simulink model "AE_BoltEV_LMDI"  (R2026a)
settings: Solver=ode23t  StartTime=0  StopTime=1800  FixedStep=Ts  MaxStep=0.01  EnableMultiTasking=on
InitFcn:
  | AE_BoltEV_LMDI_Params;
undefined symbols (not defined in the file): id_map, iq_map, Is_map, n_loss_bp, P, P_cu_map, P_iron_map, T_loss_bp, Tmax, V_oc
libraries: nesl_utility x14, fl_lib x12, autolibshared x2, sdl_lib x2, autolibmappedmotor x1, sl_discontinuities x1
(part 3 of 3)

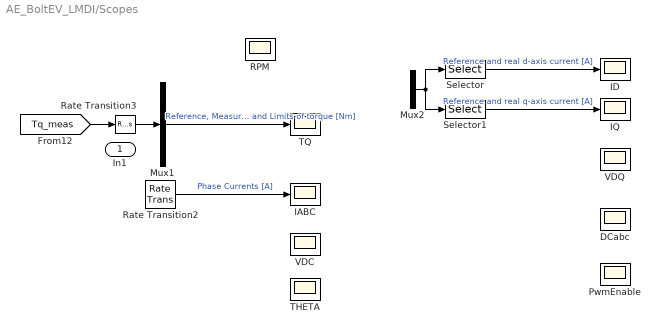
== system AE_BoltEV_LMDI/Scopes ==
  In1 : Inport
  DCabc : Scope
      settings: ActiveDisplayYMinimum=-1.2499998168622757  ActiveDisplayYMaximum=1.2499998168622755
  IABC : Scope
      settings: ActiveDisplayYMinimum=-1043.3720636046316  ActiveDisplayYMaximum=1044.7685894372053  DataLoggingVariableName=ScopeData5
  ID : Scope
      settings: ActiveDisplayYMinimum=-578.40556023238867  ActiveDisplayYMaximum=91.835041505026354  DataLoggingSaveFormat=Array
  IQ : Scope
      settings: ActiveDisplayYMinimum=-1  ActiveDisplayYMaximum=1  DataLoggingVariableName=ScopeData2  DataLoggingSaveFormat=Array
  Mux1 : Mux  Inputs=3
  Mux2 : Mux  Inputs=2
  PwmEnable : Scope
      settings: ActiveDisplayYMinimum=-0.12499999999999997  ActiveDisplayYMaximum=1.125  DataLoggingSaveFormat=Array
  RPM : Scope
      settings: ActiveDisplayYMinimum=-1  ActiveDisplayYMaximum=1
  Rate Transition2 : RateTransition  OutPortSampleTime=1e-4
  Rate Transition3 : RateTransition
  Selector : Selector  InputPortWidth=4  IndexOptions=Index vector (dialog)  Indices=[1 3]  OutputSizes=1
  Selector1 : Selector  InputPortWidth=4  IndexOptions=Index vector (dialog)  Indices=[2 4]  OutputSizes=1
  THETA : Scope
      settings: ActiveDisplayYMinimum=-0.78539816324069045  ActiveDisplayYMaximum=7.0685834691662164  DataLoggingVariableName=ScopeData7
  TQ : Scope
      settings: ActiveDisplayYMinimum=-34.876030026674364  ActiveDisplayYMaximum=3.8751144474082619  DataLoggingVariableName=ScopeData2
  VDC : Scope
      settings: ActiveDisplayYMinimum=-42.2212392731809  ActiveDisplayYMaximum=416.66871284749823  DataLoggingVariableName=ScopeData6
  VDQ : Scope
      settings: ActiveDisplayYMinimum=-252.94313596426539  ActiveDisplayYMaximum=264.44118716095903  DataLoggingVariableName=ScopeData8
  wires:
  Mux1/1 -> TQ/1  "Reference, Measured, Estim and Limits of torque [Nm]"
  Rate Transition2/1 -> IABC/1  "Phase Currents [A]"
  Selector1/1 -> IQ/1  "Reference and real q-axis current [A]"
  Selector/1 -> ID/1  "Reference and real d-axis current [A]"
  Mux2/1 -> Selector1/1, Selector/1
  [Tq_meas] -> Rate Transition3/1
  Rate Transition3/1 -> Mux1/2

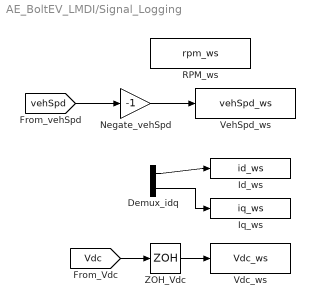
== system AE_BoltEV_LMDI/Signal_Logging ==
  Demux_idq : Demux  Outputs=2
  Id_ws : ToWorkspace  VariableName=id_ws  SampleTime=0.1
      settings: Decimation=100
  Iq_ws : ToWorkspace  VariableName=iq_ws  SampleTime=0.1
      settings: Decimation=100
  Negate_vehSpd : Gain  Gain=-1
  RPM_ws : ToWorkspace  VariableName=rpm_ws  SampleTime=0.1
      settings: Decimation=100
  Vdc_ws : ToWorkspace  VariableName=Vdc_ws  SampleTime=0.1
  VehSpd_ws : ToWorkspace  VariableName=vehSpd_ws  SampleTime=0.1
      settings: Decimation=2000
  ZOH_Vdc : ZeroOrderHold  SampleTime=0.01
  wires:
  Demux_idq/1 -> Id_ws/1
  [vehSpd] -> Negate_vehSpd/1
  ZOH_Vdc/1 -> Vdc_ws/1
  Demux_idq/2 -> Iq_ws/1
  [Vdc] -> ZOH_Vdc/1
  Negate_vehSpd/1 -> VehSpd_ws/1

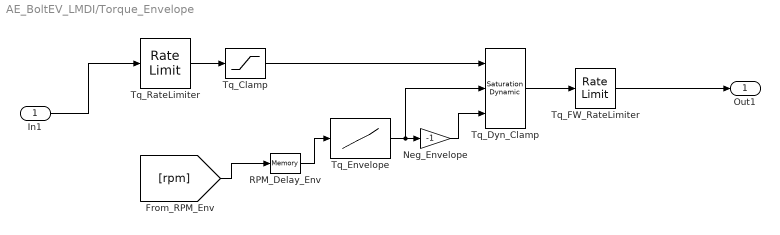
== system AE_BoltEV_LMDI/Torque_Envelope ==
  In1 : Inport
  Neg_Envelope : Gain  Gain=-1
  RPM_Delay_Env : Memory
  Tq_Clamp : Saturate  UpperLimit=Tmax  LowerLimit=-Tmax
  Tq_Dyn_Clamp : sl_discontinuities/Saturation Dynamic  OutMin=[]  OutMax=[]  OutDataTypeStr=Inherit: Same as second input  OutDataType=fixdt(1, 16)  OutScaling=2^-10  DoSatur=off
      settings: LibrarySourceBlock=|
      | simulink/Discontinuities/Saturation
      | Dynamic
  Tq_Envelope : Lookup_n-D  NumberOfTableDimensions=1  BreakpointsForDimension1=[0 1 3500 4400 5000 5500 6000 6500 7000 7500 8000 8800]  Table=[360 360 360 325 286 260 238 220 204 191 179 162]  ExtrapMethod=Clip  InternalRulePriority=Speed  RndMeth=Simplest
  Tq_FW_RateLimiter : RateLimiter  RisingSlewLimit=2000  FallingSlewLimit=-2000  SampleTimeMode=inherited
  Tq_RateLimiter : RateLimiter  RisingSlewLimit=1000  FallingSlewLimit=-1000  SampleTimeMode=inherited
  Out1 : Outport
  wires:
  In1/1 -> Tq_RateLimiter/1
  [rpm] -> RPM_Delay_Env/1
  RPM_Delay_Env/1 -> Tq_Envelope/1
  Tq_RateLimiter/1 -> Tq_Clamp/1
  Neg_Envelope/1 -> Tq_Dyn_Clamp/3
  Tq_Dyn_Clamp/1 -> Tq_FW_RateLimiter/1
  Tq_FW_RateLimiter/1 -> Out1/1
  Tq_Clamp/1 -> Tq_Dyn_Clamp/1
  Tq_Envelope/1 -> Tq_Dyn_Clamp/2, Neg_Envelope/1

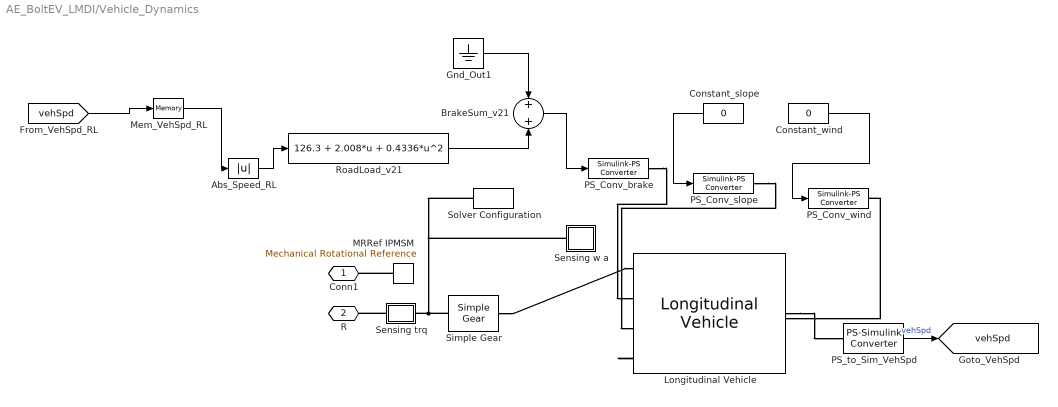
== system AE_BoltEV_LMDI/Vehicle_Dynamics ==
  Abs_Speed_RL : Abs  SaturateOnIntegerOverflow=off
  BrakeSum_v21 : Sum
  Constant_slope : Constant  Value=0
  Constant_wind : Constant  Value=0
  Gnd_Out1 : Ground
  Longitudinal Vehicle : sdl_lib/Tires & Vehicles/Longitudinal Vehicle  vehParamType=sdl.enum.VehicleParameterizationType.Regular  M_vehicle=1705 kg  R_tireroll=0.317 m  C_tireroll=1e-6  C_airdrag=1e-6  A_front=2.37 m^2  A_rl=178 N  B_rl=3.024 N*s/m  C_rl=0.36988 N*s^2/m^2  g=9.81 m/s^2  V_1=0.3 m/s  w_1=0.01 rad/s  ShowBrakeIn=true  ShowSlopeIn=true  SlopeInputType=sdl.enum.VehicleLongitudinalRoadSlopeInputType.GradePercent  ShowWindIn=true  ShowGOut=false  air_density=1.225 kg/m^3  V_x_specify=off  V_x_priority=High  V_x=0 m/s  V_x_nominal_specify=off  V_x_nominal_value=1  V_x_nominal_unit=m/s  trq_specify=off  trq_priority=None  trq=0 N*m  trq_nominal_specify=off  trq_nominal_value=1  trq_nominal_unit=N*m  w_specify=off  w_priority=None  w=0 rad/s  w_nominal_specify=off  w_nominal_value=1  w_nominal_unit=rad/s
  MRRef IPMSM : fl_lib/Mechanical/Rotational Elements/Mechanical Rotational Reference
  Mem_VehSpd_RL : Memory
  PS_Conv_brake : nesl_utility/Simulink-PS Converter  PhysicalDomain=network_engine_domain  SubClassName=ps_input  LeftPortType=input  RightPortType=output  PseudoPeriodic=off  Frequencies=[]  NoiseDistribution=none  NoiseParameters=[]  Unit=N  AffineConversion=off  FilteringAndDerivatives=provide  SimscapeFilterOrder=1  InputFilterTimeConstant=0.001  UdotUserProvided=0
  PS_Conv_slope : nesl_utility/Simulink-PS Converter  PhysicalDomain=network_engine_domain  SubClassName=ps_input  LeftPortType=input  RightPortType=output  PseudoPeriodic=off  Frequencies=[]  NoiseDistribution=none  NoiseParameters=[]  Unit=rad  AffineConversion=off  FilteringAndDerivatives=provide  SimscapeFilterOrder=1  InputFilterTimeConstant=0.001  UdotUserProvided=0
  PS_Conv_wind : nesl_utility/Simulink-PS Converter  PhysicalDomain=network_engine_domain  SubClassName=ps_input  LeftPortType=input  RightPortType=output  PseudoPeriodic=off  Frequencies=[]  NoiseDistribution=none  NoiseParameters=[]  Unit=m/s  AffineConversion=off  FilteringAndDerivatives=provide  SimscapeFilterOrder=1  InputFilterTimeConstant=0.001  UdotUserProvided=0
  PS_to_Sim_VehSpd : nesl_utility/PS-Simulink Converter  PhysicalDomain=network_engine_domain  SubClassName=ps_output  LeftPortType=input  RightPortType=output  PseudoPeriodic=off  Frequencies=[]  VectorFormat=inherit  Unit=m/s  AffineConversion=off
  RoadLoad_v21 : Fcn  Expr=126.3 + 2.008*u + 0.4336*u^2
  Sensing trq : Subsystem
      mask Display: disp('trq')
  Sensing w a : Subsystem
      mask Display: disp('w,a')
  Simple Gear : sdl_lib/Gears/Simple Gear  ratio=7.05  rotation_direction=sdl.enum.shaftOutputDirection.opposite  friction_model=sdl.enum.gear_efficiencies_load.constant  T_noload=0 N*m  T_nom=5 N*m  efficiency_nom=0.97  efficiency=gear_eff  temperature_TLU=[280, 300, 320] K  load_TLU=[1, 5, 10] N*m  efficiency_TLU=[.95, .9, .85]  efficiency_TLU2=[.85, .8, .75; .95, .9, .85; .85, .8, .7]  w_thr=0.01 rad/s  pwr_thr=0.001 W  enable_backlash=false  hardstop_model=simscape.enum.hardstop.smooth  backlash_distance=1e-3 mm  r_base=0.1 m  transition=1e-4 mm  backlash_stiffness=1e6 N/m  backlash_damping=1e3 N*s/m  coeff_rest=0.7  v_tol=0.001 m/s  f_tol=0.001 N  tau=0.1 s  mu_visc=[0 0] N*m*s/rad  thermal_mass=50 J/K  temperature_specify=off  temperature_priority=High  temperature=300 K  temperature_nominal_specify=off  temperature_nominal_value=1  temperature_nominal_unit=K  x_backlash_specify=off  x_backlash_priority=None  x_backlash=0 mm  x_backlash_nominal_specify=off  x_backlash_nominal_value=1  x_backlash_nominal_unit=mm  f_hardstop_specify=off  f_hardstop_priority=None  f_hardstop=0 N  f_hardstop_nominal_specify=off  f_hardstop_nominal_value=1  f_hardstop_nominal_unit=N  v_backlash_specify=off  v_backlash_priority=None  v_backlash=0 m/s  v_backlash_nominal_specify=off  v_backlash_nominal_value=1  v_backlash_nominal_unit=m/s
  Solver Configuration : nesl_utility/Solver Configuration  PhysicalDomain=network_engine_domain  SubClassName=solver  LeftPortType=input  RightPortType=generic  Tones=[]  Harmonics=[]  SimulateNoise=off  Profile=off  UseLocalSampling=off  EnableSwitchedLinearOptims=on  FrequencyDomain=off  UseCCode=off  RelTol=0.001  AbsTol=1e-06  MinStep=1e-09  ToWorkspace=off  RevertToSquareIcSolve=off  NumHomotopyIterations=100  PhasorMode=off  PhasorModeNumHarmonics=1  ConsistencySolver=NEWTON_FTOL  CanonicalOrdering=UNORDERED  OptimizeIntermediates=UNOPTIMIZED  IndexReductionMethod=DerivativeReplacement  DoDC=off  ResidualTolerance=1e-9  ConsistencyTolSource=GLOBAL  ConsistencyAbsTol=0.001  ConsistencyRelTol=0.001  ConsistencyTolFactor=0.001  UseLocalSolver=on  LocalSolverChoice=NE_BACKWARD_EULER_ADVANCER  ResolveIndetEquations=on  FunctionEvalNumThread=1  LocalSolverSampleTime=Ts  DoFixedCost=on  MaxNonlinIter=5  MaxModeIter=2  ComputeImpulses=off  ImpulseIterations=1  LinearAlgebra=auto  LinearAlgebraNumThread=0  EquationFormulation=NE_TIME_EF  DelaysMemoryBudget=1024  AutomaticFiltering=on  FilteringTimeConstant=0.001  PartitionStorageMethod=AS_NEEDED  PartitionMemoryBudget=1024  PartitionMethod=FAST  MultibodyUseLocalSolver=off  MultibodyLocalSolverChoice=ODE1  MultibodyLocalSolverSampleTime=0.001
  Conn1 : PMIOPort  Side=Left
  R : PMIOPort  Port=2  Side=Left
  tag scope: vehSpd=global
  wires:
  PS_to_Sim_VehSpd/1 -> [vehSpd]  "vehSpd"
  Constant_slope/1 -> PS_Conv_slope/1
  Constant_wind/1 -> PS_Conv_wind/1
  Abs_Speed_RL/1 -> RoadLoad_v21/1
  RoadLoad_v21/1 -> BrakeSum_v21/2
  BrakeSum_v21/1 -> PS_Conv_brake/1
  [vehSpd] -> Mem_VehSpd_RL/1
  Mem_VehSpd_RL/1 -> Abs_Speed_RL/1
  Gnd_Out1/1 -> BrakeSum_v21/1
  connections:
  PS_Conv_slope/RConn1 -- Longitudinal Vehicle/LConn3
  PS_Conv_brake/RConn1 -- Longitudinal Vehicle/LConn2
  Sensing trq/LConn1 -- R/RConn1
  Longitudinal Vehicle/RConn1 -- PS_to_Sim_VehSpd/LConn1
  Simple Gear/RConn1 -- Longitudinal Vehicle/LConn1
  MRRef IPMSM/LConn1 -- Conn1/RConn1
  Longitudinal Vehicle/LConn4 -- PS_Conv_wind/RConn1
  Simple Gear/LConn1 -- Sensing w a/LConn1 -- Solver Configuration/RConn1 -- Sensing trq/RConn1

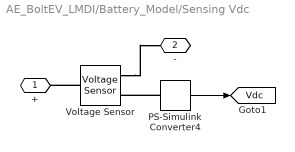
== system AE_BoltEV_LMDI/Battery_Model/Sensing Vdc ==
  PS-Simulink Converter4 : nesl_utility/PS-Simulink Converter  PhysicalDomain=network_engine_domain  SubClassName=ps_output  LeftPortType=input  RightPortType=output  PseudoPeriodic=off  Frequencies=[]  VectorFormat=1-D array  Unit=V  AffineConversion=off
  Voltage Sensor : fl_lib/Electrical/Electrical Sensors/Voltage Sensor
  + : PMIOPort  Side=Left
  - : PMIOPort  Port=2  Side=Right
  tag scope: Vdc=global
  wires:
  PS-Simulink Converter4/1 -> [Vdc]
  connections:
  Voltage Sensor/LConn1 -- +/RConn1
  Voltage Sensor/RConn2 -- -/RConn1
  PS-Simulink Converter4/LConn1 -- Voltage Sensor/RConn1

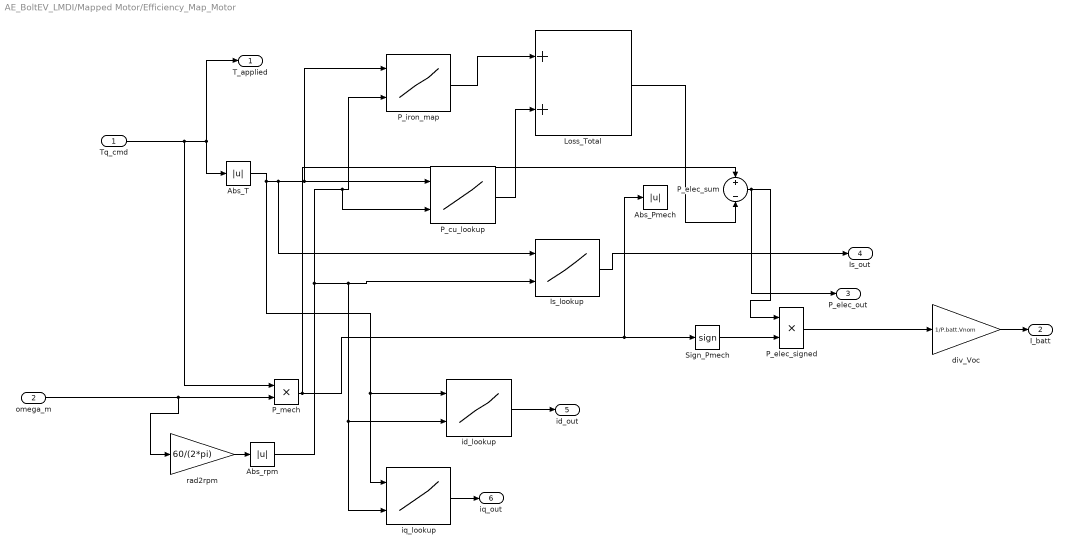
== system AE_BoltEV_LMDI/Mapped Motor/Efficiency_Map_Motor ==
  Tq_cmd : Inport
  omega_m : Inport  Port=2
  Abs_Pmech : Abs
  Abs_T : Abs
  Abs_rpm : Abs
  Is_lookup : Lookup_n-D  BreakpointsForDimension1=T_loss_bp  BreakpointsForDimension2=n_loss_bp  Table=Is_map  ExtrapMethod=Clip  InternalRulePriority=Speed  RndMeth=Simplest
      settings: InputPortMap=u0,u1
  Loss_Total : Sum
  P_cu_lookup : Lookup_n-D  BreakpointsForDimension1=T_loss_bp  BreakpointsForDimension2=n_loss_bp  Table=P_cu_map  ExtrapMethod=Clip  InternalRulePriority=Speed  RndMeth=Simplest
      settings: InputPortMap=u0,u1
  P_elec_signed : Product
  P_elec_sum : Sum  Inputs=+-
  P_iron_map : Lookup_n-D  BreakpointsForDimension1=T_loss_bp  BreakpointsForDimension2=n_loss_bp  Table=P_iron_map  ExtrapMethod=Clip  InternalRulePriority=Speed  RndMeth=Simplest
      settings: InputPortMap=u0,u1
  P_mech : Product
  Sign_Pmech : Signum
  div_Voc : Gain  Gain=1/P.batt.Vnom
  id_lookup : Lookup_n-D  BreakpointsForDimension1=T_loss_bp  BreakpointsForDimension2=n_loss_bp  Table=id_map  ExtrapMethod=Clip  InternalRulePriority=Speed  RndMeth=Simplest
      settings: InputPortMap=u0,u1
  iq_lookup : Lookup_n-D  BreakpointsForDimension1=T_loss_bp  BreakpointsForDimension2=n_loss_bp  Table=iq_map  ExtrapMethod=Clip  InternalRulePriority=Speed  RndMeth=Simplest
      settings: InputPortMap=u0,u1
  rad2rpm : Gain  Gain=60/(2*pi)
  T_applied : Outport
  I_batt : Outport  Port=2
  P_elec_out : Outport  Port=3
  Is_out : Outport  Port=4
  id_out : Outport  Port=5
  iq_out : Outport  Port=6
  wires:
  Tq_cmd/1 -> Abs_T/1, T_applied/1, P_mech/1
  omega_m/1 -> rad2rpm/1, P_mech/2
  rad2rpm/1 -> Abs_rpm/1
  Abs_T/1 -> id_lookup/1, iq_lookup/1, P_iron_map/1, P_cu_lookup/1, Is_lookup/1
  Abs_rpm/1 -> P_iron_map/2, P_cu_lookup/2, Is_lookup/2, iq_lookup/2, id_lookup/2
  P_mech/1 -> Abs_Pmech/1, Sign_Pmech/1, P_elec_sum/1
  P_elec_sum/1 -> P_elec_signed/1, P_elec_out/1
  Sign_Pmech/1 -> P_elec_signed/2
  P_elec_signed/1 -> div_Voc/1
  div_Voc/1 -> I_batt/1
  P_iron_map/1 -> Loss_Total/1
  P_cu_lookup/1 -> Loss_Total/2
  Loss_Total/1 -> P_elec_sum/2
  Is_lookup/1 -> Is_out/1
  id_lookup/1 -> id_out/1
  iq_lookup/1 -> iq_out/1

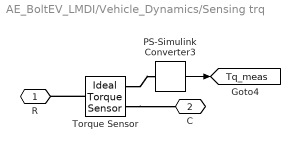
== system AE_BoltEV_LMDI/Vehicle_Dynamics/Sensing trq ==
  PS-Simulink Converter3 : nesl_utility/PS-Simulink Converter  PhysicalDomain=network_engine_domain  SubClassName=ps_output  LeftPortType=input  RightPortType=output  PseudoPeriodic=off  Frequencies=[]  VectorFormat=1-D array  Unit=N*m  AffineConversion=off
  Torque Sensor : fl_lib/Mechanical/Mechanical Sensors/Ideal Torque Sensor
  R : PMIOPort  Side=Left
  C : PMIOPort  Port=2  Side=Right
  tag scope: Tq_meas=global
  wires:
  PS-Simulink Converter3/1 -> [Tq_meas]
  connections:
  Torque Sensor/RConn1 -- C/RConn1
  Torque Sensor/RConn2 -- PS-Simulink Converter3/LConn1
  Torque Sensor/LConn1 -- R/RConn1

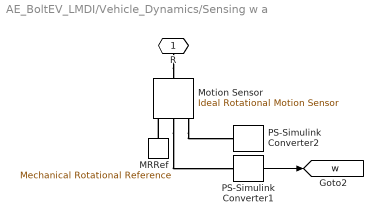
== system AE_BoltEV_LMDI/Vehicle_Dynamics/Sensing w a ==
  MRRef : fl_lib/Mechanical/Rotational Elements/Mechanical Rotational Reference
  Motion Sensor : fl_lib/Mechanical/Mechanical Sensors/Ideal Rotational Motion Sensor  reference=foundation.enum.MeasurementReference.difference  acceleration_port=false  velocity_port=true  position_port=true  wrap_angle=simscape.enum.onoff.off  offset=0 deg
  PS-Simulink Converter1 : nesl_utility/PS-Simulink Converter  PhysicalDomain=network_engine_domain  SubClassName=ps_output  LeftPortType=input  RightPortType=output  PseudoPeriodic=off  Frequencies=[]  VectorFormat=1-D array  Unit=rad/s  AffineConversion=off
  PS-Simulink Converter2 : nesl_utility/PS-Simulink Converter  PhysicalDomain=network_engine_domain  SubClassName=ps_output  LeftPortType=input  RightPortType=output  PseudoPeriodic=off  Frequencies=[]  VectorFormat=1-D array  Unit=rad  AffineConversion=off
  R : PMIOPort  Side=Left
  tag scope: w=global
  wires:
  PS-Simulink Converter1/1 -> [w]
  connections:
  R/RConn1 -- Motion Sensor/LConn1
  Motion Sensor/RConn2 -- PS-Simulink Converter1/LConn1
  MRRef/LConn1 -- Motion Sensor/RConn1
  Motion Sensor/RConn3 -- PS-Simulink Converter2/LConn1
